simulink model "rfpsc_grid"  (R2023b)
settings: Solver=VariableStepAuto  StartTime=0.0  StopTime=.5  RelTol=1e-3
undefined symbols (not defined in the file): f_sw, K_p, L_f, L_g, R_a, R_L, T_s, U_dc, u_gN, w_b, w_g
libraries: simulink x1
settings Model: Creator=maatt  LastModifiedBy=maatt
settings DataIOCC: ReturnWorkspaceOutputs=off

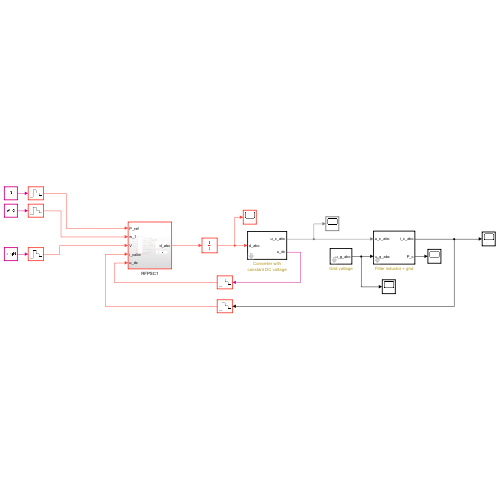
[thumbnail: Simulink's stored preview of the top-level diagram]
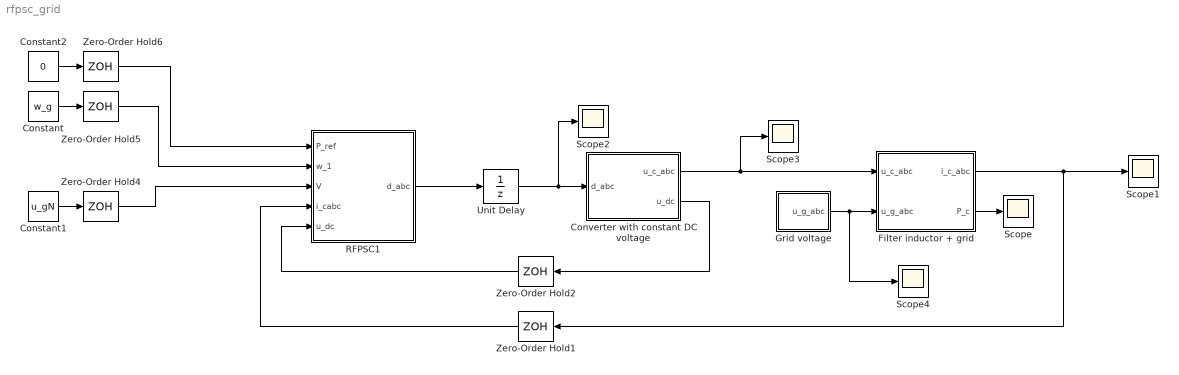
== system rfpsc_grid ==
  Constant : Constant  Value=w_g
  Constant1 : Constant  Value=u_gN
  Constant2 : Constant  Value=0
  "Converter with constant DC voltage " : Subsystem  mask{f_sw=f_sw, u_dc=U_dc}
      mask prompts: f_sw "Switching frequency (Hz)"; u_dc "DC-bus voltage (V)"
      mask init:
      | T_s = 1/(2*f_sw);
  Filter inductor + grid : Subsystem  mask{L_f=L_f, L_g=L_g, R_L=R_L}
      mask prompts: L_f "Filter inductance (H)"; L_g "Grid inductance (H)"; R_L "Series resistance (ohm)"
  Grid voltage : Subsystem  mask{w_g=2*pi*50, U_g=24}
      mask prompts: w_g "Grid angular frequency (rad/s)"; U_g "Line-to-neutral peak voltage (V)"
  RFPSC1 : Subsystem
  Scope{,1..4} (5 alike) : Scope
  Unit Delay : UnitDelay  SampleTime=T_s  HasFrameUpgradeWarning=on
  Zero-Order Hold{1..2,4..6} (5 alike) : ZeroOrderHold  SampleTime=T_s
  wires:
  "Converter with constant DC voltage "/1(u_c_abc) -> Scope3/1, Filter inductor + grid/1(u_c_abc)
  RFPSC1/1(d_abc) -> Unit Delay/1
  "Converter with constant DC voltage "/2(u_dc) -> Zero-Order Hold2/1
  Constant/1 -> Zero-Order Hold5/1
  Constant1/1 -> Zero-Order Hold4/1
  Filter inductor + grid/1(i_c_abc) -> Scope1/1, Zero-Order Hold1/1
  Unit Delay/1 -> "Converter with constant DC voltage "/1(d_abc), Scope2/1
  Zero-Order Hold1/1 -> RFPSC1/4(i_cabc)
  Zero-Order Hold4/1 -> RFPSC1/3(V)
  Zero-Order Hold5/1 -> RFPSC1/2(w_1)
  Zero-Order Hold6/1 -> RFPSC1/1(P_ref)
  Zero-Order Hold2/1 -> RFPSC1/5(u_dc)
  Constant2/1 -> Zero-Order Hold6/1
  Grid voltage/1(u_g_abc) -> Scope4/1, Filter inductor + grid/2(u_g_abc)
  Filter inductor + grid/2(P_c) -> Scope/1

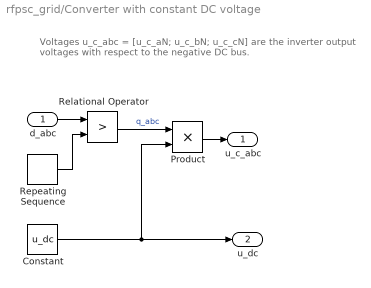
== system rfpsc_grid/Converter with constant DC voltage  ==
  note: Voltages u_c_abc = [u_c_aN; u_c_bN; u_c_cN] are the inverter
      | output voltages with respect to the negative DC bus.
  d_abc : Inport
  Constant : Constant  Value=u_dc
  Product : Product
  Relational Operator : RelationalOperator  Operator=>  OutDataTypeStr='double'  InputSameDT=off
  Repeating Sequence : simulink/Sources/Repeating Sequence  rep_seq_t=[0 1 2]*T_s  rep_seq_y=[1 0 1]
  u_c_abc : Outport
  u_dc : Outport  Port=2
  wires:
  Repeating Sequence/1 -> Relational Operator/2
  d_abc/1 -> Relational Operator/1
  Product/1 -> u_c_abc/1
  Relational Operator/1 -> Product/1  "q_abc"
  Constant/1 -> Product/2, u_dc/1

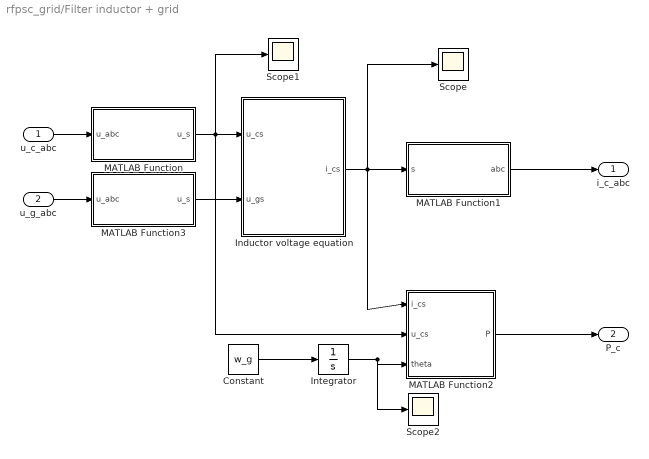
== system rfpsc_grid/Filter inductor + grid ==
  u_c_abc : Inport
  u_g_abc : Inport  Port=2
  Constant : Constant  Value=w_g
  Inductor voltage equation : Subsystem
  Integrator : Integrator  WrapState=on
  MATLAB Function : MATLAB Function  TreatAsAtomicUnit=on
  MATLAB Function1 : MATLAB Function  TreatAsAtomicUnit=on
  MATLAB Function2 : MATLAB Function  TreatAsAtomicUnit=on
  MATLAB Function3 : MATLAB Function  TreatAsAtomicUnit=on
  Scope : Scope
  Scope1 : Scope
  Scope2 : Scope
  i_c_abc : Outport
  P_c : Outport  Port=2
  wires:
  u_c_abc/1 -> MATLAB Function/1(u_abc)
  MATLAB Function/1(u_s) -> Scope1/1, MATLAB Function2/2(u_cs), Inductor voltage equation/1(u_cs)
  u_g_abc/1 -> MATLAB Function3/1(u_abc)
  MATLAB Function3/1(u_s) -> Inductor voltage equation/2(u_gs)
  Inductor voltage equation/1(i_cs) -> Scope/1, MATLAB Function2/1(i_cs), MATLAB Function1/1(s)
  MATLAB Function1/1(abc) -> i_c_abc/1
  Constant/1 -> Integrator/1
  Integrator/1 -> Scope2/1, MATLAB Function2/3(theta)
  MATLAB Function2/1(P) -> P_c/1

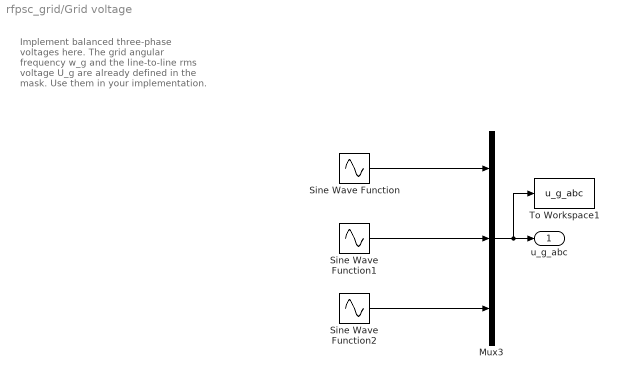
== system rfpsc_grid/Grid voltage ==
  note: Implement balanced three-phase
      | voltages here. The grid angular
      | frequency w_g and the line-to-line rms
      | voltage U_g are already defined
      | in the mask. Use them in your
      | implementation.
  Mux3 : Mux  Inputs=3
  Sine Wave Function : Sin  Amplitude=U_g  Frequency=w_g
  Sine Wave Function1 : Sin  Amplitude=U_g  Frequency=w_g  Phase=2*pi/3
  Sine Wave Function2 : Sin  Amplitude=U_g  Frequency=w_g  Phase=4*pi/3
  To Workspace1 : ToWorkspace  VariableName=u_g_abc  SaveFormat=Timeseries  SampleTime=-1
  u_g_abc : Outport
  wires:
  Mux3/1 -> To Workspace1/1, u_g_abc/1
  Sine Wave Function/1 -> Mux3/1
  Sine Wave Function1/1 -> Mux3/2
  Sine Wave Function2/1 -> Mux3/3

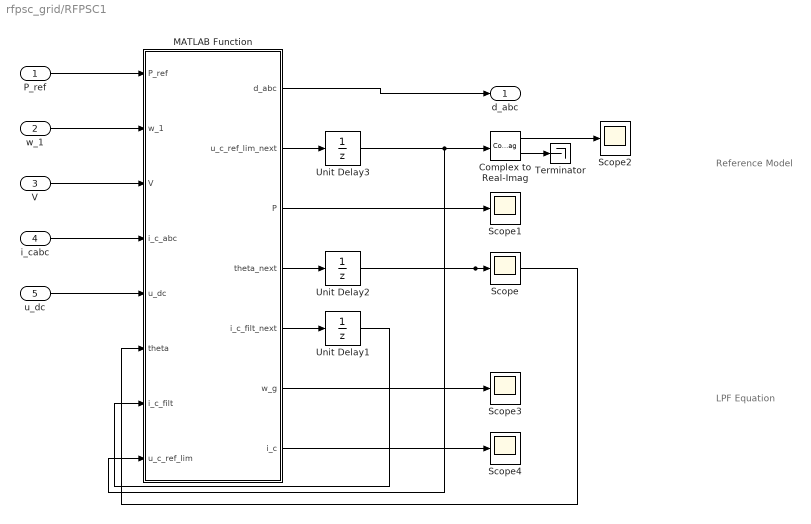
== system rfpsc_grid/RFPSC1 ==
  note: Reference Model
  note: LPF Equation
  P_ref : Inport
  w_1 : Inport  Port=2
  V : Inport  Port=3
  i_cabc : Inport  Port=4
  u_dc : Inport  Port=5
  Complex to Real-Imag : ComplexToRealImag
  MATLAB Function : MATLAB Function  TreatAsAtomicUnit=on
  Scope{,1..4} (5 alike) : Scope
  Terminator : Terminator
  Unit Delay1 : UnitDelay  SampleTime=-1  HasFrameUpgradeWarning=on
  Unit Delay2 : UnitDelay  SampleTime=-1  HasFrameUpgradeWarning=on
  Unit Delay3 : UnitDelay  SampleTime=-1  HasFrameUpgradeWarning=on
  d_abc : Outport
  wires:
  P_ref/1 -> MATLAB Function/1(P_ref)
  w_1/1 -> MATLAB Function/2(w_1)
  V/1 -> MATLAB Function/3(V)
  i_cabc/1 -> MATLAB Function/4(i_c_abc)
  MATLAB Function/1(d_abc) -> d_abc/1
  MATLAB Function/5(i_c_filt_next) -> Unit Delay1/1
  Unit Delay1/1 -> MATLAB Function/7(i_c_filt)
  MATLAB Function/4(theta_next) -> Unit Delay2/1
  Unit Delay2/1 -> MATLAB Function/6(theta), Scope/1
  u_dc/1 -> MATLAB Function/5(u_dc)
  MATLAB Function/2(u_c_ref_lim_next) -> Unit Delay3/1
  MATLAB Function/3(P) -> Scope1/1
  Unit Delay3/1 -> Complex to Real-Imag/1, MATLAB Function/8(u_c_ref_lim)
  MATLAB Function/6(w_g) -> Scope3/1
  Complex to Real-Imag/1 -> Scope2/1
  Complex to Real-Imag/2 -> Terminator/1
  MATLAB Function/7(i_c) -> Scope4/1

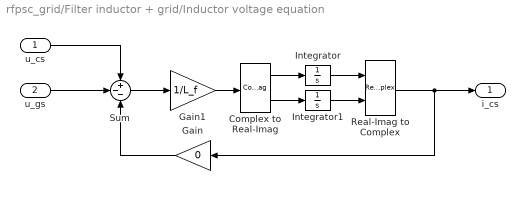
== system rfpsc_grid/Filter inductor + grid/Inductor voltage equation ==
  u_cs : Inport
  u_gs : Inport  Port=2
  Complex to Real-Imag : ComplexToRealImag
  Gain : Gain  Gain=0
  Gain1 : Gain  Gain=1/L_f
  Integrator : Integrator
  Integrator1 : Integrator
  Real-Imag to Complex : RealImagToComplex
  Sum : Sum  Inputs=+--
  i_cs : Outport
  wires:
  Real-Imag to Complex/1 -> Gain/1, i_cs/1
  Gain/1 -> Sum/3
  Sum/1 -> Gain1/1
  u_gs/1 -> Sum/2
  Gain1/1 -> Complex to Real-Imag/1
  u_cs/1 -> Sum/1
  Integrator/1 -> Real-Imag to Complex/1
  Complex to Real-Imag/1 -> Integrator/1
  Complex to Real-Imag/2 -> Integrator1/1
  Integrator1/1 -> Real-Imag to Complex/2

== matlab function rfpsc_grid/RFPSC1/MATLAB Function ==
  data: P_ref input; d_abc output; u_c_ref_lim_next output; P output; theta_next output; w_1 input; V input; i_c_abc input; u_dc input; theta input; i_c_filt input; K_p parameter; T_s parameter; R_a parameter; i_c_filt_next output; w_b parameter; u_c_ref_lim input; w_g output; i_c output
function [d_abc, u_c_ref_lim_next, P, theta_next, i_c_filt_next, w_g, i_c] = RFPSC(P_ref, w_1, V, i_c_abc, u_dc,...
   theta, i_c_filt, K_p, T_s, R_a, w_b, u_c_ref_lim)

% Space Vector Transformation of converter current (abcTos)
i_cs = 2/3*(i_c_abc(1) + i_c_abc(2)*exp(1j*2*pi/3) + i_c_abc(3)*exp(1j*4*pi/3));

% Coordinate transformation of converter current
i_c = i_cs*exp(-1j*theta);

% Active power calculation
P = 3/2*real(u_c_ref_lim*conj(i_c));

% Equation for grid angular frequency
w_g = (P_ref - P)*K_p + w_1;

% Update (integrate) the grid voltage angle
theta_next = theta + 1.5 * T_s * w_g; % Discrete time compensation
while(theta_next > pi)
    theta_next = theta_next - 2*pi;
end
while(theta_next < -pi)
    theta_next = theta_next + 2*pi;
end

% Extracting the real and imaginary values of the complex converter current
i_c_imag = imag(i_c);

% Applying lowpass filter equation to imaginary part of the
% converter current and forming reference current based on power reference
i_c_filt_next =  i_c_filt*(1 - w_b*T_s) + i_c_imag*(w_b*T_s);
i_ref = P_ref/V + 1j*i_c_filt_next;

% Equation for reference voltage
u_c = V + (i_ref-i_c) * R_a;

% Inverse coordinate transformation
u_cs_ref = u_c*exp(1j*theta);


%% Symmetrical suboscillation PWM
% Components of the voltage space vector
u_c_alpha_ref = real(u_cs_ref);
u_c_beta_ref  = imag(u_cs_ref);

% Phase-voltage references
u_ca_ref = u_c_alpha_ref;
u_cb_ref = .5*(-u_c_alpha_ref + sqrt(3)*u_c_beta_ref);
u_cc_ref = .5*(-u_c_alpha_ref - sqrt(3)*u_c_beta_ref);

% Vector of phase-voltage references
u_c_abc_ref = [u_ca_ref; u_cb_ref; u_cc_ref];

% Symmetrization of the references by adding the zero-sequence voltage
u0 = .5*(max(u_c_abc_ref) + min(u_c_abc_ref));
u_c_abc_ref = u_c_abc_ref - u0;

% Clipping of the reference voltages such that no phase error is caused. 
% If all phase voltage reference are realizable (below u_dc/2), m = 1 holds.
m = max([2*u_c_abc_ref/u_dc; 1]);
u_c_abc_ref = u_c_abc_ref/m;

% Duty cycles, which can be directly used for triangle comparison, 
% if the triangle wave varies between 0...1
d_abc = .5 + u_c_abc_ref/u_dc;
% 
% % Realized voltage vector is calculated from the clamped duty ratios.
% % If the PWM does not saturate, u_c_ref_lim = u_c_ref holds. The realized
% % voltage vector is needed, e.g., for the current-controller antiwindup.
u_cs_ref_lim = 2/3*(d_abc(1) + d_abc(2)*exp(1j*2*pi/3) ...
     + d_abc(3)*exp(1j*4*pi/3))*u_dc;
% % In estimated rotor flux coordinates
u_c_ref_lim_next = exp(-1j*theta_next)*u_cs_ref_lim;

== matlab function rfpsc_grid/Filter inductor + grid/MATLAB Function3 ==
  data: u_abc input size=3; u_s output size=1
function u_s = abc2s(u_abc)

% Space-vector transformation
u_s = 2/3*(u_abc(1) + u_abc(2)*exp(1j*2*pi/3) + u_abc(3)*exp(1j*4*pi/3));

== matlab function rfpsc_grid/Filter inductor + grid/MATLAB Function1 ==
  data: s input size=1; abc output size=3
function abc = s2abc(s)

% Inverse space-vector transformation
abc = real([1; exp(-1j*2*pi/3); exp(-1j*4*pi/3)]*s);

== matlab function rfpsc_grid/Filter inductor + grid/MATLAB Function2 ==
  data: i_cs input; P output; u_cs input; theta input
function P = fcn(i_cs, u_cs, theta)

% Coordinate transformation
i_c = i_cs*exp(-1j*theta);
u_c = u_cs*exp(-1j*theta);

% Active power calculation
P = 3/2*real(u_c*conj(i_c));

== matlab function rfpsc_grid/Filter inductor + grid/MATLAB Function ==
  data: u_abc input size=3; u_s output size=1
function u_s = abc2s(u_abc)

% Space-vector transformation
u_s = 2/3*(u_abc(1) + u_abc(2)*exp(1j*2*pi/3) + u_abc(3)*exp(1j*4*pi/3));
